simulink model "compare_pst_kapa_tau"  (R2020b)
settings: Solver=VariableStepAuto  StartTime=0.0  StopTime=150  RelTol=1e-3
values from neighbouring files (symbols this model uses):
  c_kap = 0.4    [lab4.m]
  c_tau = 0.3    [lab4.m]
  tf_kap = td_kap / N_kap    [lab4.m]
  tf_tau = td_tau / N_tau    [lab4.m]
  tt_kap = sqrt(ti_kap+td_kap)    [lab4.m]
  tt_tau = sqrt(ti_tau+td_tau)    [lab4.m]
undefined symbols (not defined in the file or in its folder): b_kap, b_tau, kp_kap, kp_tau, plant_1, td_kap, td_tau, ti_kap, ti_tau
settings Model: Creator=user1  LastModifiedBy=rafael
settings SFSimCC: CustomCodeUndefinedFunction=UseInterfaceOnly

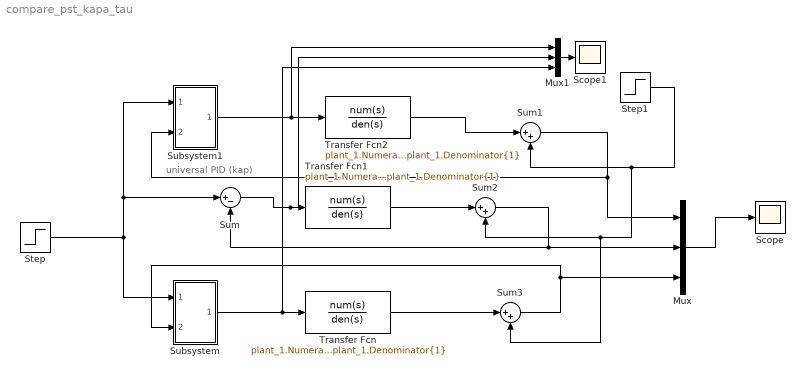
== system compare_pst_kapa_tau ==
  note: universal PID (kap)
  Mux : Mux  Inputs=3
  Mux1 : Mux  Inputs=3
  Scope : Scope
  Scope1 : Scope
  Step : Step  SampleTime=0
  Step1 : Step  Time=80  SampleTime=0
  Subsystem : Subsystem
  Subsystem1 : Subsystem
  Sum : Sum  Inputs=|+-
  Sum1 : Sum  Inputs=|++
  Sum2 : Sum  Inputs=|++
  Sum3 : Sum  Inputs=|++
  Transfer Fcn : TransferFcn  Numerator=plant_1.Numerator{1}  Denominator=plant_1.Denominator{1}
  Transfer Fcn1 : TransferFcn  Numerator=plant_1.Numerator{1}  Denominator=plant_1.Denominator{1}
  Transfer Fcn2 : TransferFcn  Numerator=plant_1.Numerator{1}  Denominator=plant_1.Denominator{1}
  wires:
  Step/1 -> Subsystem1/1(In1), Sum/1, Subsystem/1(In1)
  Subsystem/1(Out1) -> Mux1/3, Transfer Fcn/1
  Mux/1 -> Scope/1
  Sum/1 -> Mux1/2, Transfer Fcn1/1
  Subsystem1/1(Out1) -> Mux1/1, Transfer Fcn2/1
  Mux1/1 -> Scope1/1
  Step1/1 -> Sum3/2, Sum2/2, Sum1/2
  Transfer Fcn2/1 -> Sum1/1
  Sum1/1 -> Mux/1, Subsystem1/2(In2)
  Transfer Fcn/1 -> Sum3/1
  Transfer Fcn1/1 -> Sum2/1
  Sum3/1 -> Subsystem/2(In2), Mux/3
  Sum2/1 -> Mux/2, Sum/2

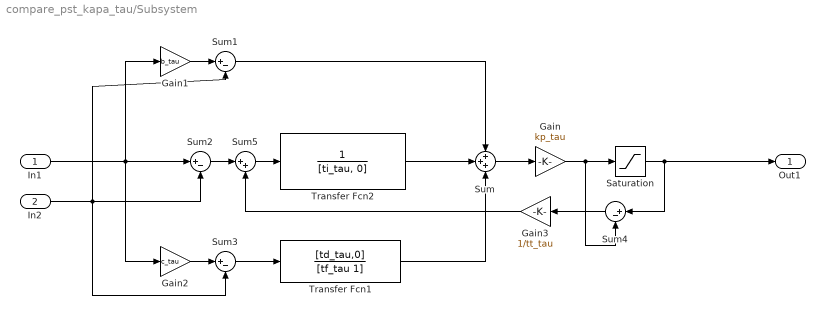
== system compare_pst_kapa_tau/Subsystem ==
  In1 : Inport
  In2 : Inport  Port=2
  Gain : Gain  Gain=kp_tau
  Gain1 : Gain  Gain=b_tau
  Gain2 : Gain  Gain=c_tau
  Gain3 : Gain  Gain=1/tt_tau
  Saturation : Saturate  UpperLimit=1  LowerLimit=-1
  Sum : Sum  Inputs=+++
  Sum{1..4} (4 alike) : Sum  Inputs=|+-
  Sum5 : Sum  Inputs=|++
  Transfer Fcn1 : TransferFcn  Numerator=[td_tau,0]  Denominator=[tf_tau 1]
  Transfer Fcn2 : TransferFcn  Denominator=[ti_tau, 0]
  Out1 : Outport  VectorParamsAs1DForOutWhenUnconnected=off
  wires:
  Transfer Fcn1/1 -> Sum/3
  In1/1 -> Gain2/1, Sum2/1, Gain1/1
  Sum/1 -> Gain/1
  Gain2/1 -> Sum3/1
  In2/1 -> Sum2/2, Sum3/2, Sum1/2
  Sum1/1 -> Sum/1
  Sum3/1 -> Transfer Fcn1/1
  Gain1/1 -> Sum1/1
  Gain/1 -> Sum4/2, Saturation/1
  Sum4/1 -> Gain3/1
  Gain3/1 -> Sum5/2
  Sum2/1 -> Sum5/1
  Sum5/1 -> Transfer Fcn2/1
  Transfer Fcn2/1 -> Sum/2
  Saturation/1 -> Out1/1, Sum4/1

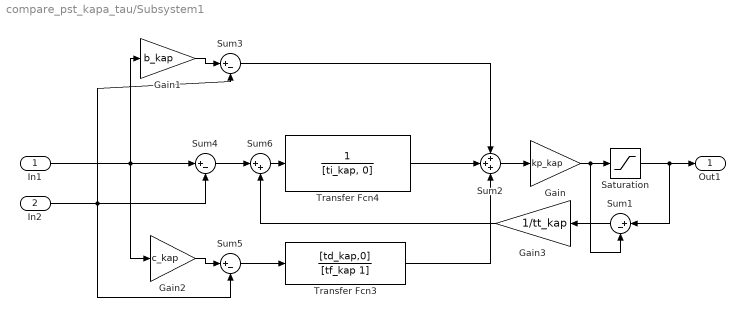
== system compare_pst_kapa_tau/Subsystem1 ==
  In1 : Inport
  In2 : Inport  Port=2
  Gain : Gain  Gain=kp_kap
  Gain1 : Gain  Gain=b_kap
  Gain2 : Gain  Gain=c_kap
  Gain3 : Gain  Gain=1/tt_kap
  Saturation : Saturate  UpperLimit=1  LowerLimit=-1
  Sum{1,3..5} (4 alike) : Sum  Inputs=|+-
  Sum2 : Sum  Inputs=+++
  Sum6 : Sum  Inputs=|++
  Transfer Fcn3 : TransferFcn  Numerator=[td_kap,0]  Denominator=[tf_kap 1]
  Transfer Fcn4 : TransferFcn  Denominator=[ti_kap, 0]
  Out1 : Outport  VectorParamsAs1DForOutWhenUnconnected=off
  wires:
  In2/1 -> Sum4/2, Sum5/2, Sum3/2
  Transfer Fcn3/1 -> Sum2/3
  Gain2/1 -> Sum5/1
  In1/1 -> Gain2/1, Sum4/1, Gain1/1
  Sum3/1 -> Sum2/1
  Sum2/1 -> Gain/1
  Sum5/1 -> Transfer Fcn3/1
  Gain1/1 -> Sum3/1
  Transfer Fcn4/1 -> Sum2/2
  Gain/1 -> Sum1/2, Saturation/1
  Saturation/1 -> Sum1/1, Out1/1
  Sum1/1 -> Gain3/1
  Gain3/1 -> Sum6/2
  Sum4/1 -> Sum6/1
  Sum6/1 -> Transfer Fcn4/1
